simulink library "INP_SPR"  (R2024b)
settings: Solver=VariableStepAuto  StartTime=0.0  StopTime=10.0  RelTol=1e-3
libraries: INP_SPR_ManOver x1, INP_SPR_Prep x1
settings Model: Creator=blatak  LastModifiedBy=jmbsp

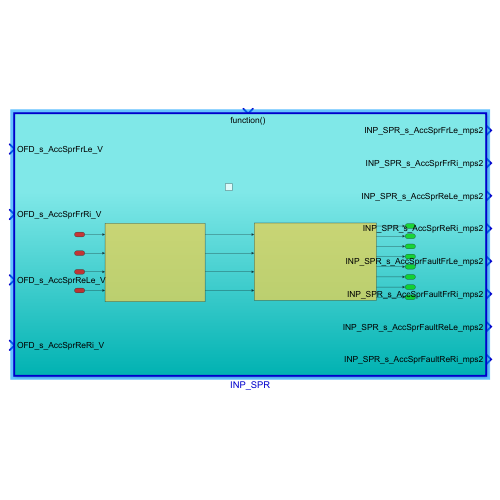
[thumbnail: Simulink's stored preview of the top-level diagram]
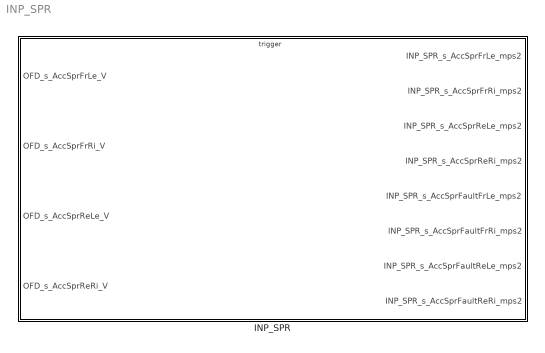
== system INP_SPR ==
  INP_SPR : Subsystem  TreatAsAtomicUnit=on

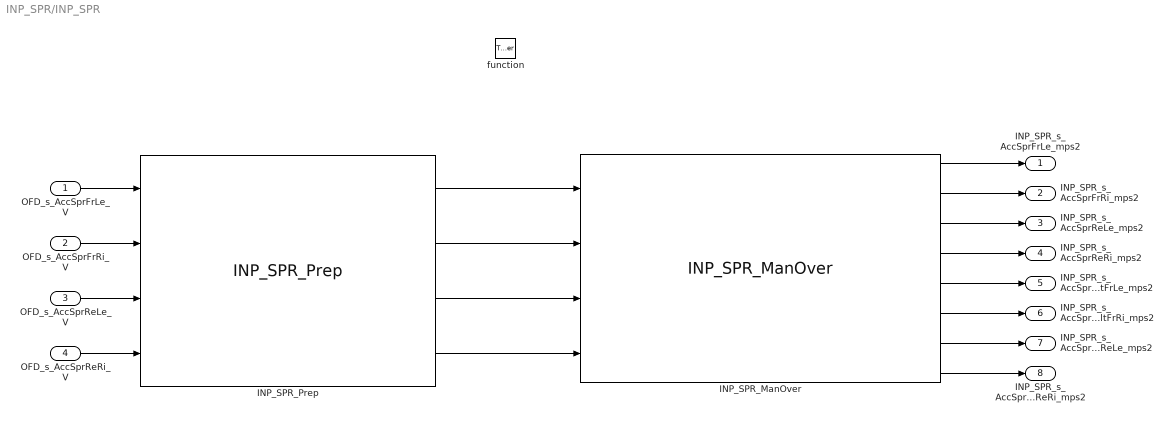
== system INP_SPR/INP_SPR ==
  OFD_s_AccSprFrLe_V : Inport
  OFD_s_AccSprFrRi_V : Inport  Port=2
  OFD_s_AccSprReLe_V : Inport  Port=3
  OFD_s_AccSprReRi_V : Inport  Port=4
  function : TriggerPort  TriggerType=function-call  VariantControl=(inherit)
  INP_SPR_ManOver : INP_SPR_ManOver/INP_SPR_ManOver  SystemSampleTime=-1  VariantActivationTime=update diagram  AllowFlexibleInterface=on  Latency=0  AutoFrameSizeCalculation=off
  INP_SPR_Prep : INP_SPR_Prep/INP_SPR_Prep  SystemSampleTime=-1  VariantActivationTime=update diagram  AllowFlexibleInterface=on  Latency=0  AutoFrameSizeCalculation=off
  INP_SPR_s_AccSprFrLe_mps2 : Outport
  INP_SPR_s_AccSprFrRi_mps2 : Outport  Port=2
  INP_SPR_s_AccSprReLe_mps2 : Outport  Port=3
  INP_SPR_s_AccSprReRi_mps2 : Outport  Port=4
  INP_SPR_s_AccSprFaultFrLe_mps2 : Outport  Port=5
  INP_SPR_s_AccSprFaultFrRi_mps2 : Outport  Port=6
  INP_SPR_s_AccSprFaultReLe_mps2 : Outport  Port=7
  INP_SPR_s_AccSprFaultReRi_mps2 : Outport  Port=8
  wires:
  INP_SPR_Prep/1 -> INP_SPR_ManOver/1
  INP_SPR_Prep/2 -> INP_SPR_ManOver/2
  INP_SPR_Prep/3 -> INP_SPR_ManOver/3
  INP_SPR_Prep/4 -> INP_SPR_ManOver/4
  OFD_s_AccSprFrLe_V/1 -> INP_SPR_Prep/1
  OFD_s_AccSprFrRi_V/1 -> INP_SPR_Prep/2
  OFD_s_AccSprReLe_V/1 -> INP_SPR_Prep/3
  OFD_s_AccSprReRi_V/1 -> INP_SPR_Prep/4
  INP_SPR_ManOver/1 -> INP_SPR_s_AccSprFrLe_mps2/1
  INP_SPR_ManOver/2 -> INP_SPR_s_AccSprFrRi_mps2/1
  INP_SPR_ManOver/3 -> INP_SPR_s_AccSprReLe_mps2/1
  INP_SPR_ManOver/4 -> INP_SPR_s_AccSprReRi_mps2/1
  INP_SPR_ManOver/5 -> INP_SPR_s_AccSprFaultFrLe_mps2/1
  INP_SPR_ManOver/6 -> INP_SPR_s_AccSprFaultFrRi_mps2/1
  INP_SPR_ManOver/7 -> INP_SPR_s_AccSprFaultReLe_mps2/1
  INP_SPR_ManOver/8 -> INP_SPR_s_AccSprFaultReRi_mps2/1
